simulink model "uavsimblockset_trimModel_Cularis_turbulentAtmosphere"  (Simulink 8.6)
settings: Solver=ode45  StartTime=0.0  StopTime=1  FixedStep=1/30  RelTol=1e-3
undefined symbols (not defined in the file): Earth, uavsim, WGS84
libraries: aerolibadyn x2, uavsimBlockset_DerivedAerodynamicConditions x1, uavsimBlockset_ElectricPropulsion x1, aerolibobsolete x1, aerolibtransform2 x1, uavsimblockset_vbody2vNED x1, aerolibgravity2 x1, uavsimBlockset_VectorNorm x1
settings Model: Creator=mstolle  LastModifiedBy=j.bolting
settings SolverCC: AutoInsertRateTranBlk=on
settings DataIOCC: SignalLoggingSaveFormat=Dataset
settings DebuggingCC: SolverPrmCheckMsg=none  FcnCallInpInsideContextMsg=EnableAllAsError  BusObjectLabelMismatch=error
settings ModelReferenceCC: ModelReferenceMinAlgLoopOccurrences=on
settings GRTTargetCC: CombineOutputUpdateFcns=on  GRTInterface=off
settings ConfigComp: CovSFcnEnable=off

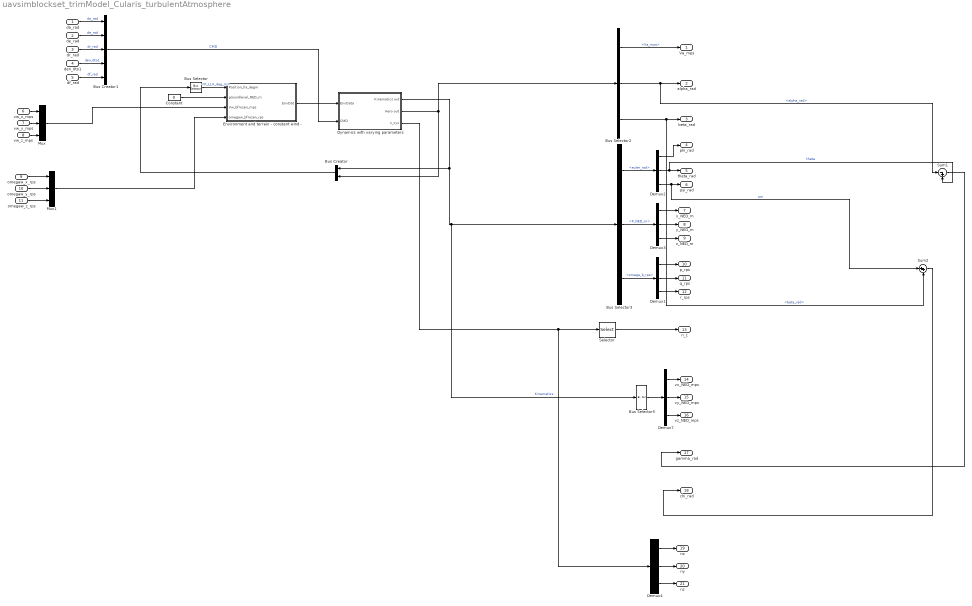
== system uavsimblockset_trimModel_Cularis_turbulentAtmosphere ==
  da_rad : Inport
  de_rad : Inport  Port=2
  dr_rad : Inport  Port=3
  den_0to1 : Inport  Port=4
  df_rad : Inport  Port=5
  vw_x_mps : Inport  Port=6  PortDimensions=1
  vw_y_mps : Inport  Port=7  PortDimensions=1
  vw_z_mps : Inport  Port=8  PortDimensions=1
  omegaw_x_rps : Inport  Port=9  PortDimensions=1
  omegaw_y_rps : Inport  Port=10  PortDimensions=1
  omegaw_z_rps : Inport  Port=11  PortDimensions=1
  Bus Creator1 : BusCreator  Inputs=5  OutDataTypeStr=Bus: CMD  NonVirtualBus=on
  Bus Creator : BusCreator  Inputs=2
  Bus Selector : BusSelector  OutputSignals=Kinematics.Position.P_LLA_deg_m
  Bus Selector2 : BusSelector  OutputSignals=Va_mps,alpha_rad,beta_rad
  Bus Selector3 : BusSelector  OutputSignals=Attitude.euler_rad,Position.P_NED_m,RotationalVelocity.omega_b_rps
  Bus Selector5 : BusSelector  OutputSignals=Velocity.Vground_NED_mps  OutputAsBus=on
  Constant : Constant  Value=0
  Demux{1..4,7} (5 alike) : Demux  Outputs=3
  Dynamics with varying parameters : Subsystem  mask{uavsim=uavsim}
      mask prompts: uavsim "Parameter structure"
  Environment and terrain - constant wind - : Subsystem  AncestorBlock=uavsimBlockset_Environment_calmAtmosphere/Environment and terrain - calm atmosphere -
  Mux : Mux  Inputs=3
  Mux1 : Mux  Inputs=3
  Selector : Selector  InputPortWidth=3  IndexOptions=Index vector (dialog)  Indices=1  OutputSizes=1
  Sum1 : Sum  Inputs=|-+
  Sum2 : Sum  Inputs=|++
  Va_mps : Outport
  alpha_rad : Outport  Port=2
  beta_rad : Outport  Port=3
  phi_rad : Outport  Port=4
  theta_rad : Outport  Port=5
  psi_rad : Outport  Port=6
  x_NED_m : Outport  Port=7
  y_NED_m : Outport  Port=8
  z_NED_m : Outport  Port=9
  p_rps : Outport  Port=10
  q_rps : Outport  Port=11
  r_rps : Outport  Port=12
  n_z : Outport  Port=13
  vx_NED_mps : Outport  Port=14
  vy_NED_mps : Outport  Port=15
  vz_NED_mps : Outport  Port=16
  gamma_rad : Outport  Port=17
  chi_rad : Outport  Port=18
  nx : Outport  Port=19
  ny : Outport  Port=20
  nz : Outport  Port=21
  wires:
  den_0to1/1 -> Bus Creator1/4  "den_0to1"
  de_rad/1 -> Bus Creator1/2  "de_rad"
  da_rad/1 -> Bus Creator1/1  "da_rad"
  dr_rad/1 -> Bus Creator1/3  "dr_rad"
  Bus Creator1/1 -> Dynamics with varying parameters/2(CMD)  "CMD"
  Environment and terrain - constant wind -/1(EnvDat) -> Dynamics with varying parameters/1(EnvData)
  df_rad/1 -> Bus Creator1/5  "df_rad"
  Bus Creator/1 -> Bus Selector/1
  Constant/1 -> Environment and terrain - constant wind -/2(groundlevel_NED_m)
  Bus Selector/1 -> Environment and terrain - constant wind -/1(Position_lla_degm)  "<P_LLA_deg_m>"
  Mux/1 -> Environment and terrain - constant wind -/3(Vw_bfrozen_mps)
  Mux1/1 -> Environment and terrain - constant wind -/4(omegaw_bfrozen_rps)
  Dynamics with varying parameters/2(Aero out) -> Bus Creator/2, Bus Selector2/1
  vw_z_mps/1 -> Mux/3
  vw_y_mps/1 -> Mux/2
  vw_x_mps/1 -> Mux/1
  omegaw_x_rps/1 -> Mux1/1
  omegaw_z_rps/1 -> Mux1/3
  omegaw_y_rps/1 -> Mux1/2
  Bus Selector3/1 -> Demux2/1  "<euler_rad>"
  Demux2/1 -> phi_rad/1
  Bus Selector3/3 -> Demux1/1  "<omega_b_rps>"
  Demux1/1 -> p_rps/1
  Demux1/2 -> q_rps/1
  Demux1/3 -> r_rps/1
  Bus Selector2/1 -> Va_mps/1  "<Va_mps>"
  Bus Selector3/2 -> Demux3/1  "<P_NED_m>"
  Demux3/1 -> x_NED_m/1
  Demux3/2 -> y_NED_m/1
  Demux3/3 -> z_NED_m/1
  Dynamics with varying parameters/3(n_xyz) -> Demux4/1, Selector/1
  Dynamics with varying parameters/1(Kinematics out) -> Bus Selector5/1, Bus Selector3/1, Bus Creator/1  "Kinematics"
  Bus Selector5/1 -> Demux7/1
  Bus Selector2/3 -> Sum2/2, beta_rad/1  "<beta_rad>"
  Bus Selector2/2 -> Sum1/1, alpha_rad/1  "<alpha_rad>"
  Demux2/2 -> theta_rad/1, Sum1/2  "theta"
  Sum1/1 -> gamma_rad/1
  Demux2/3 -> Sum2/1, psi_rad/1  "psi"
  Sum2/1 -> chi_rad/1
  Demux7/1 -> vx_NED_mps/1
  Demux7/2 -> vy_NED_mps/1
  Demux7/3 -> vz_NED_mps/1
  Selector/1 -> n_z/1
  Demux4/1 -> nx/1
  Demux4/2 -> ny/1
  Demux4/3 -> nz/1

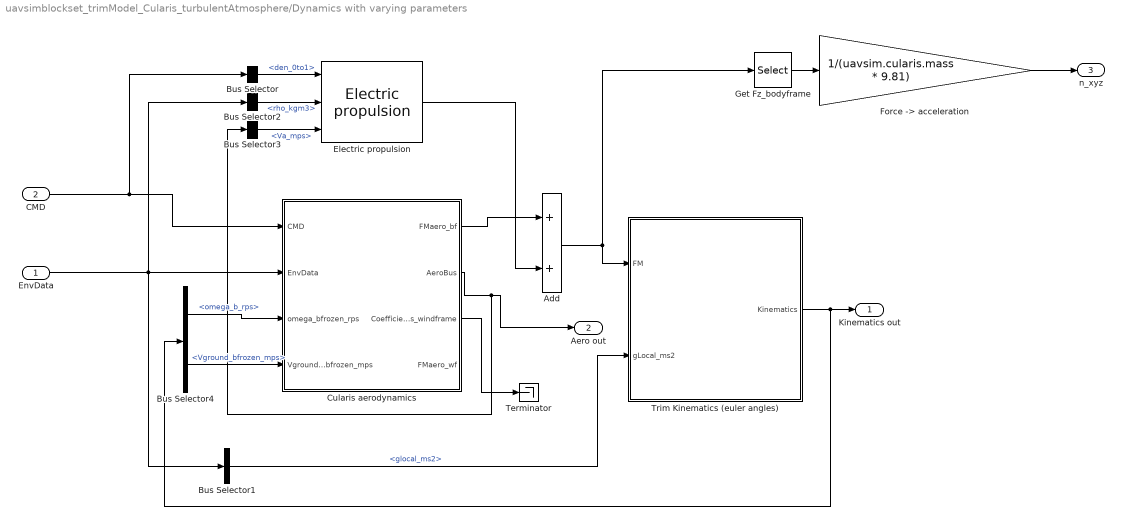
== system uavsimblockset_trimModel_Cularis_turbulentAtmosphere/Dynamics with varying parameters ==
  EnvData : Inport  OutDataTypeStr=Bus: Environment
  CMD : Inport  Port=2  OutDataTypeStr=Bus: CMD
  Add : Sum
  Bus Selector : BusSelector  OutputSignals=den_0to1
  Bus Selector1 : BusSelector  OutputSignals=glocal_ms2
  Bus Selector2 : BusSelector  OutputSignals=rho_kgm3
  Bus Selector3 : BusSelector  OutputSignals=Va_mps
  Bus Selector4 : BusSelector  OutputSignals=RotationalVelocity.omega_b_rps,Velocity.Vground_bfrozen_mps
  Cularis aerodynamics : Subsystem  AncestorBlock=uavsimBlockset_Cularis_Aerandpropulsion/Cularis aerodynamics
  Electric propulsion : uavsimBlockset_ElectricPropulsion/Electric propulsion  mask_C_prop=uavsim.cularis.C_prop  mask_S_prop=uavsim.cularis.S_prop  mask_k_motor=uavsim.cularis.k_motor
  "Force -> acceleration" : Gain  Gain=1/(uavsim.cularis.mass * 9.81)
  Get Fz_bodyframe : Selector  InputPortWidth=6  IndexOptions=Index vector (dialog)  Indices=1:3  OutputSizes=1
  Terminator : Terminator
  Trim Kinematics (euler angles) : Subsystem  AncestorBlock=uavsimblockset_TrimKinematics/Trim Kinematics (euler angles)  mask{mask_inertia=uavsim.cularis.inertiaTensor, mask_mass=uavsim.cularis.mass, mask_P0_ECEF_m=uavsim.mojaveairport_ecef_m, mask_uvw0=[15 0 0], mask_phithetapsi0=[0 0 0], mask_omega0=[0 0 0]}
      mask prompts: mask_inertia "Inertia tensor [kg * m²]"; mask_mass "Aircraft mass [kg]"; mask_P0_ECEF_m "Initial ECEF position [m]"; mask_uvw0 "Initial velocity vector, body frame [m/s]"; mask_phithetapsi0 "Initial Euler angles [rad]"; mask_omega0 "Initial body rotation rates [rad/s]"
  Kinematics out : Outport  OutDataTypeStr=Bus: Kinematics
  Aero out : Outport  Port=2  OutDataTypeStr=Bus: Aero
  n_xyz : Outport  Port=3  PortDimensions=3
  wires:
  Bus Selector4/2 -> Cularis aerodynamics/4(Vground_bfrozen_mps)  "<Vground_bfrozen_mps>"
  Bus Selector4/1 -> Cularis aerodynamics/3(omega_bfrozen_rps)  "<omega_b_rps>"
  Trim Kinematics (euler angles)/1(Kinematics) -> Kinematics out/1, Bus Selector4/1
  EnvData/1 -> Bus Selector2/1, Bus Selector1/1, Cularis aerodynamics/2(EnvData)
  Add/1 -> Get Fz_bodyframe/1, Trim Kinematics (euler angles)/1(FM)
  Cularis aerodynamics/1(FMaero_bf) -> Add/1
  Cularis aerodynamics/3(Coefficients_windframe) -> Terminator/1
  Bus Selector1/1 -> Trim Kinematics (euler angles)/2(gLocal_ms2)  "<glocal_ms2>"
  Get Fz_bodyframe/1 -> "Force -> acceleration"/1
  "Force -> acceleration"/1 -> n_xyz/1
  Bus Selector/1 -> Electric propulsion/1  "<den_0to1>"
  Bus Selector3/1 -> Electric propulsion/3  "<Va_mps>"
  Bus Selector2/1 -> Electric propulsion/2  "<rho_kgm3>"
  CMD/1 -> Bus Selector/1, Cularis aerodynamics/1(CMD)
  Cularis aerodynamics/2(AeroBus) -> Bus Selector3/1, Aero out/1
  Electric propulsion/1 -> Add/2

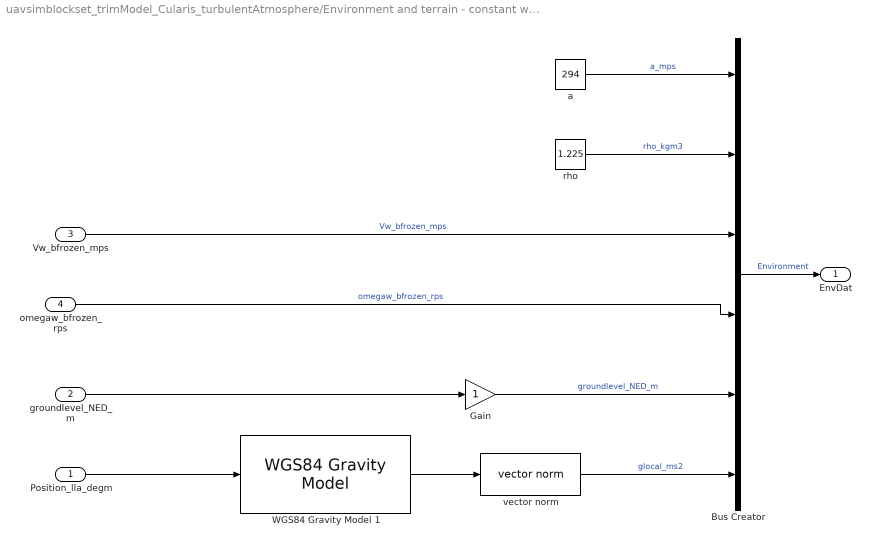
== system uavsimblockset_trimModel_Cularis_turbulentAtmosphere/Environment and terrain - constant wind - ==
  Position_lla_degm : Inport
  groundlevel_NED_m : Inport  Port=2
  Vw_bfrozen_mps : Inport  Port=3
  omegaw_bfrozen_rps : Inport  Port=4
  Bus Creator : BusCreator  Inputs=6  OutDataTypeStr=Bus: Environment  NonVirtualBus=on
  Gain : Gain
  WGS84 Gravity Model 1 : aerolibgravity2/WGS84 Gravity Model   model=WGS84 Taylor Series  units=Metric (MKS)  no_atmos=on  precessing=on  jd_loc=off  month=October  day=10  year=2004  no_centrifugal=on  action=Warning
  a : Constant  Value=294
  "rho " : Constant  Value=1.225
  vector norm : uavsimBlockset_VectorNorm/vector norm
  EnvDat : Outport  OutDataTypeStr=Bus: Environment
  wires:
  Gain/1 -> Bus Creator/5  "groundlevel_NED_m"
  omegaw_bfrozen_rps/1 -> Bus Creator/4  "omegaw_bfrozen_rps"
  vector norm/1 -> Bus Creator/6  "glocal_ms2"
  Vw_bfrozen_mps/1 -> Bus Creator/3  "Vw_bfrozen_mps"
  a/1 -> Bus Creator/1  "a_mps"
  "rho "/1 -> Bus Creator/2  "rho_kgm3"
  Bus Creator/1 -> EnvDat/1  "Environment"
  WGS84 Gravity Model 1/1 -> vector norm/1
  groundlevel_NED_m/1 -> Gain/1
  Position_lla_degm/1 -> WGS84 Gravity Model 1/1

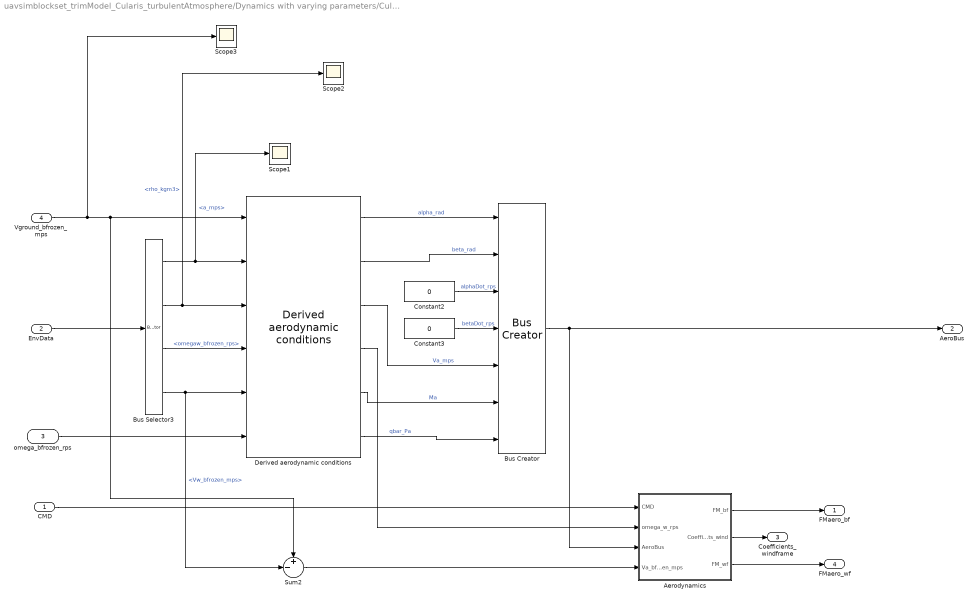
== system uavsimblockset_trimModel_Cularis_turbulentAtmosphere/Dynamics with varying parameters/Cularis aerodynamics ==
  CMD : Inport  OutDataTypeStr=Bus: CMD
  EnvData : Inport  Port=2  OutDataTypeStr=Bus: Environment
  omega_bfrozen_rps : Inport  Port=3
  Vground_bfrozen_mps : Inport  Port=4
  Aerodynamics : Subsystem
  Bus Selector3 : BusSelector  OutputSignals=a_mps,rho_kgm3,omegaw_bfrozen_rps,Vw_bfrozen_mps
  Bus Creator : BusCreator  Inputs=7
  Constant2 : Constant  Value=0
  Constant3 : Constant  Value=0
  Derived aerodynamic conditions : uavsimBlockset_DerivedAerodynamicConditions/Derived aerodynamic conditions
  Scope1 : Scope
  Scope2 : Scope
  Scope3 : Scope
  Sum2 : Sum  Inputs=+-|  SaturateOnIntegerOverflow=on  InputSameDT=on  OutDataTypeStr=Inherit: Same as first input
  FMaero_bf : Outport
  AeroBus : Outport  Port=2  OutDataTypeStr=Bus: Aero
  Coefficients_windframe : Outport  Port=3
  FMaero_wf : Outport  Port=4
  wires:
  Derived aerodynamic conditions/4 -> Aerodynamics/2(omega_w_rps)
  Sum2/1 -> Aerodynamics/4(Va_bfrozen_mps)
  Bus Creator/1 -> Aerodynamics/3(AeroBus), AeroBus/1
  Derived aerodynamic conditions/6 -> Bus Creator/7  "qbar_Pa"
  Derived aerodynamic conditions/5 -> Bus Creator/6  "Ma"
  Derived aerodynamic conditions/3 -> Bus Creator/5  "Va_mps"
  Derived aerodynamic conditions/2 -> Bus Creator/2  "beta_rad"
  Derived aerodynamic conditions/1 -> Bus Creator/1  "alpha_rad"
  Vground_bfrozen_mps/1 -> Scope3/1, Derived aerodynamic conditions/1, Sum2/1
  Constant3/1 -> Bus Creator/4  "betaDot_rps"
  Constant2/1 -> Bus Creator/3  "alphaDot_rps"
  Bus Selector3/4 -> Sum2/2, Derived aerodynamic conditions/5  "<Vw_bfrozen_mps>"
  Bus Selector3/3 -> Derived aerodynamic conditions/4  "<omegaw_bfrozen_rps>"
  Bus Selector3/2 -> Scope2/1, Derived aerodynamic conditions/3  "<rho_kgm3>"
  Bus Selector3/1 -> Scope1/1, Derived aerodynamic conditions/2  "<a_mps>"
  Aerodynamics/2(Coefficients_wind) -> Coefficients_windframe/1
  CMD/1 -> Aerodynamics/1(CMD)
  Aerodynamics/1(FM_bf) -> FMaero_bf/1
  omega_bfrozen_rps/1 -> Derived aerodynamic conditions/6
  EnvData/1 -> Bus Selector3/1
  Aerodynamics/3(FM_wf) -> FMaero_wf/1

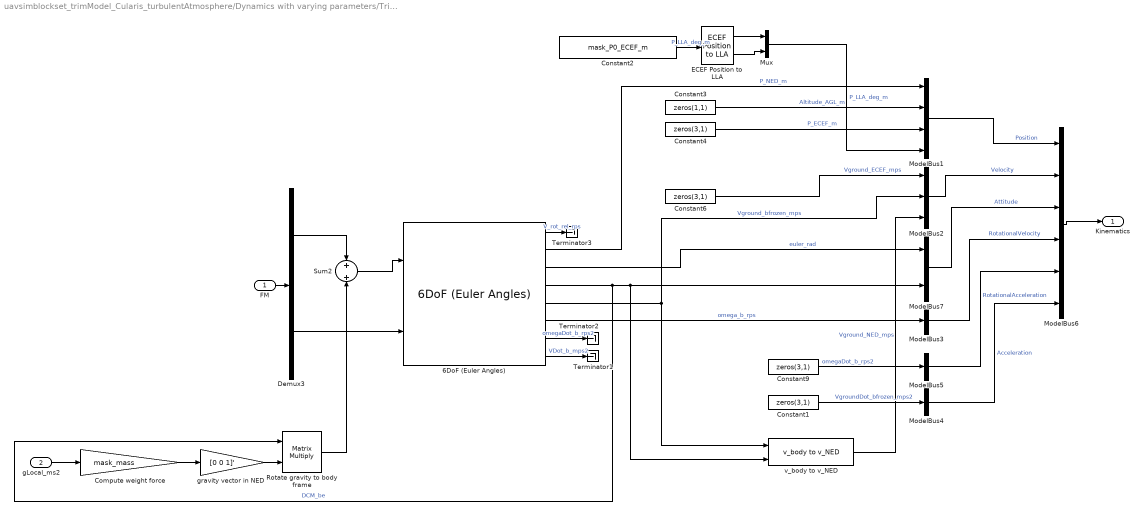
== system uavsimblockset_trimModel_Cularis_turbulentAtmosphere/Dynamics with varying parameters/Trim Kinematics (euler angles) ==
  FM : Inport
  gLocal_ms2 : Inport  Port=2
  6DoF (Euler Angles) : aerolibobsolete/6DoF (Euler Angles)  units=Metric (MKS)  mtype=Fixed  rep=Euler Angles  xme_0=mask_P0_ECEF_m  Vm_0=mask_uvw0  eul_0=mask_phithetapsi0  pm_0=mask_omega0  mass_0=mask_mass  mass_e=0.5  mass_f=2.0  inertia=mask_inertia  inertia_e=eye(3)  inertia_f=2*eye(3)  k_quat=1.0
  Compute weight force : Gain  Gain=mask_mass
  Constant{1,4,6,9} (4 alike) : Constant  Value=zeros(3,1)  SampleTime=-1
  Constant2 : Constant  Value=mask_P0_ECEF_m  SampleTime=-1
  Constant3 : Constant  Value=zeros(1,1)  SampleTime=-1
  Demux3 : Demux  Outputs=[3,3]
  ECEF Position to LLA : aerolibtransform2/ECEF Position to LLA  units=Metric (MKS)  ptype=Earth (WGS84)  F=1/298.257223563  R=6378137
  ModelBus1 : BusCreator  Inputs='P_NED_m','Altitude_AGL_m','P_ECEF_m','P_LLA_deg_m'  OutDataTypeStr=Bus: Position  NonVirtualBus=on
  ModelBus2 : BusCreator  Inputs=3  OutDataTypeStr=Bus: Velocity  NonVirtualBus=on
  ModelBus3 : BusCreator  Inputs='omega_b_rps'  OutDataTypeStr=Bus: RotationalVelocity  NonVirtualBus=on
  ModelBus4 : BusCreator  Inputs=1  OutDataTypeStr=Bus: Acceleration  NonVirtualBus=on
  ModelBus5 : BusCreator  Inputs='omegaDot_b_rps2'  OutDataTypeStr=Bus: RotationalAcceleration  NonVirtualBus=on
  ModelBus6 : BusCreator  Inputs=6  OutDataTypeStr=Bus: Kinematics
  ModelBus7 : BusCreator  Inputs='euler_rad','DCM_be'  OutDataTypeStr=Bus: Attitude  NonVirtualBus=on
  Mux : Mux  Inputs=2
  Rotate gravity to body frame : Product  Multiplication=Matrix(*)
  Sum2 : Sum  SaturateOnIntegerOverflow=on  InputSameDT=on  OutDataTypeStr=Inherit: Same as first input
  Terminator1 : Terminator
  Terminator2 : Terminator
  Terminator3 : Terminator
  gravity vector in NED : Gain  Gain=[0 0 1]'
  v_body to v_NED : uavsimblockset_vbody2vNED/v_body to v_NED
  Kinematics : Outport  OutDataTypeStr=Bus: Kinematics
  wires:
  ECEF Position to LLA/2 -> Mux/2
  ECEF Position to LLA/1 -> Mux/1
  Constant2/1 -> ECEF Position to LLA/1  "P_LLA_deg_m"
  Rotate gravity to body frame/1 -> Sum2/2
  Compute weight force/1 -> gravity vector in NED/1
  gravity vector in NED/1 -> Rotate gravity to body frame/2
  gLocal_ms2/1 -> Compute weight force/1
  v_body to v_NED/1 -> ModelBus2/3  "Vground_NED_mps"
  6DoF (Euler Angles)/1 -> Terminator3/1  "V_rot_rel_rps"
  FM/1 -> Demux3/1
  Constant9/1 -> ModelBus5/1  "omegaDot_b_rps2"
  6DoF (Euler Angles)/7 -> Terminator2/1  "omegaDot_b_rps2"
  6DoF (Euler Angles)/8 -> Terminator1/1  "VDot_b_mps2"
  Constant1/1 -> ModelBus4/1  "VgroundDot_bfrozen_mps2"
  ModelBus6/1 -> Kinematics/1
  6DoF (Euler Angles)/5 -> v_body to v_NED/1, ModelBus2/2  "Vground_bfrozen_mps"
  6DoF (Euler Angles)/2 -> ModelBus1/1  "P_NED_m"
  Mux/1 -> ModelBus1/4  "P_LLA_deg_m"
  Constant3/1 -> ModelBus1/2  "Altitude_AGL_m"
  ModelBus5/1 -> ModelBus6/5  "RotationalAcceleration"
  ModelBus2/1 -> ModelBus6/2  "Velocity"
  ModelBus3/1 -> ModelBus6/4  "RotationalVelocity"
  6DoF (Euler Angles)/3 -> ModelBus7/1  "euler_rad"
  Constant6/1 -> ModelBus2/1  "Vground_ECEF_mps"
  Demux3/2 -> 6DoF (Euler Angles)/2
  Sum2/1 -> 6DoF (Euler Angles)/1
  6DoF (Euler Angles)/6 -> ModelBus3/1  "omega_b_rps"
  6DoF (Euler Angles)/4 -> ModelBus7/2, v_body to v_NED/2, Rotate gravity to body frame/1  "DCM_be"
  Demux3/1 -> Sum2/1
  ModelBus7/1 -> ModelBus6/3  "Attitude"
  Constant4/1 -> ModelBus1/3  "P_ECEF_m"
  ModelBus1/1 -> ModelBus6/1  "Position"
  ModelBus4/1 -> ModelBus6/6  "Acceleration"

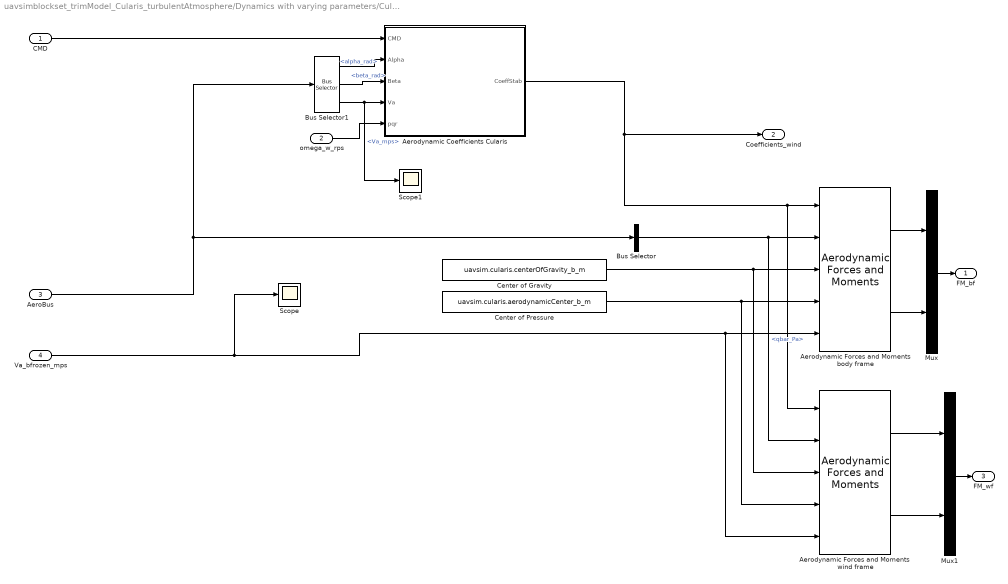
== system uavsimblockset_trimModel_Cularis_turbulentAtmosphere/Dynamics with varying parameters/Cularis aerodynamics/Aerodynamics ==
  CMD : Inport  OutDataTypeStr=Bus: CMD
  omega_w_rps : Inport  Port=2
  AeroBus : Inport  Port=3  OutDataTypeStr=Bus: Aero
  Va_bfrozen_mps : Inport  Port=4
  Aerodynamic Coefficients Cularis : Subsystem
  "Aerodynamic Forces and Moments body frame " : aerolibadyn/Aerodynamic Forces and Moments   inputAxes=Wind  outputForceAxes=Body  outputMomentAxes=Body  S=uavsim.cularis.S  b=uavsim.cularis.b  cbar=uavsim.cularis.c
  Aerodynamic Forces and Moments  wind frame : aerolibadyn/Aerodynamic Forces and Moments   inputAxes=Wind  outputForceAxes=Wind  outputMomentAxes=Wind  S=uavsim.cularis.S  b=uavsim.cularis.b  cbar=uavsim.cularis.c
  Bus Selector1 : BusSelector  OutputSignals=alpha_rad,beta_rad,Va_mps
  Bus Selector : BusSelector  OutputSignals=qbar_Pa
  Center of Gravity : Constant  Value=uavsim.cularis.centerOfGravity_b_m  SampleTime=0
  Center of Pressure : Constant  Value=uavsim.cularis.aerodynamicCenter_b_m  SampleTime=0
  Mux : Mux  Inputs=2
  Mux1 : Mux  Inputs=2
  Scope : Scope
  Scope1 : Scope
  FM_bf : Outport
  Coefficients_wind : Outport  Port=2
  FM_wf : Outport  Port=3
  wires:
  Va_bfrozen_mps/1 -> Scope/1, Aerodynamic Forces and Moments  wind frame/5, "Aerodynamic Forces and Moments body frame "/5
  omega_w_rps/1 -> Aerodynamic Coefficients Cularis/5(pqr)
  Bus Selector1/3 -> Scope1/1, Aerodynamic Coefficients Cularis/4(Va)  "<Va_mps>"
  Bus Selector1/2 -> Aerodynamic Coefficients Cularis/3(Beta)  "<beta_rad>"
  Bus Selector1/1 -> Aerodynamic Coefficients Cularis/2(Alpha)  "<alpha_rad>"
  AeroBus/1 -> Bus Selector1/1, Bus Selector/1
  Bus Selector/1 -> Aerodynamic Forces and Moments  wind frame/2, "Aerodynamic Forces and Moments body frame "/2  "<qbar_Pa>"
  Mux/1 -> FM_bf/1
  CMD/1 -> Aerodynamic Coefficients Cularis/1(CMD)
  Center of Pressure/1 -> Aerodynamic Forces and Moments  wind frame/4, "Aerodynamic Forces and Moments body frame "/4
  Center of Gravity/1 -> Aerodynamic Forces and Moments  wind frame/3, "Aerodynamic Forces and Moments body frame "/3
  "Aerodynamic Forces and Moments body frame "/1 -> Mux/1
  Aerodynamic Coefficients Cularis/1(CoeffStab) -> Coefficients_wind/1, "Aerodynamic Forces and Moments body frame "/1, Aerodynamic Forces and Moments  wind frame/1
  "Aerodynamic Forces and Moments body frame "/2 -> Mux/2
  Mux1/1 -> FM_wf/1
  Aerodynamic Forces and Moments  wind frame/1 -> Mux1/1
  Aerodynamic Forces and Moments  wind frame/2 -> Mux1/2

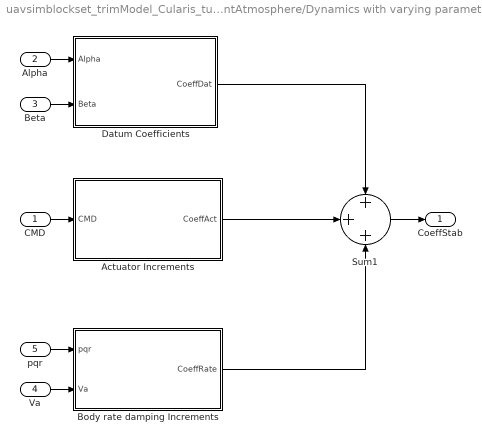
== system uavsimblockset_trimModel_Cularis_turbulentAtmosphere/Dynamics with varying parameters/Cularis aerodynamics/Aerodynamics/Aerodynamic Coefficients Cularis ==
  CMD : Inport
  Alpha : Inport  Port=2
  Beta : Inport  Port=3
  Va : Inport  Port=4
  pqr : Inport  Port=5
  Actuator Increments : Subsystem
  Body rate damping Increments : Subsystem
  Datum Coefficients : Subsystem
  Sum1 : Sum  Inputs=+++  SaturateOnIntegerOverflow=on  InputSameDT=on  OutDataTypeStr=Inherit: Same as first input
  CoeffStab : Outport
  wires:
  Datum Coefficients/1(CoeffDat) -> Sum1/1
  Sum1/1 -> CoeffStab/1
  CMD/1 -> Actuator Increments/1(CMD)
  Beta/1 -> Datum Coefficients/2(Beta)
  pqr/1 -> Body rate damping Increments/1(pqr)
  Va/1 -> Body rate damping Increments/2(Va)
  Alpha/1 -> Datum Coefficients/1(Alpha)
  Body rate damping Increments/1(CoeffRate) -> Sum1/3
  Actuator Increments/1(CoeffAct) -> Sum1/2

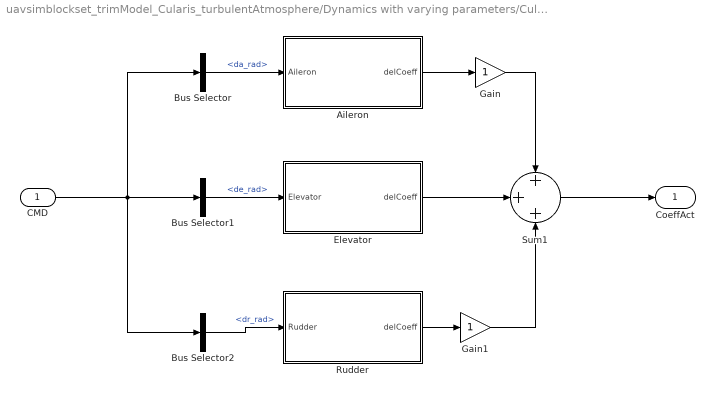
== system uavsimblockset_trimModel_Cularis_turbulentAtmosphere/Dynamics with varying parameters/Cularis aerodynamics/Aerodynamics/Aerodynamic Coefficients Cularis/Actuator Increments ==
  CMD : Inport
  Aileron : Subsystem
  Bus Selector : BusSelector  OutputSignals=da_rad
  Bus Selector1 : BusSelector  OutputSignals=de_rad
  Bus Selector2 : BusSelector  OutputSignals=dr_rad
  Elevator : Subsystem
  Gain : Gain
  Gain1 : Gain
  Rudder : Subsystem
  Sum1 : Sum  Inputs=+++  SaturateOnIntegerOverflow=on  InputSameDT=on  OutDataTypeStr=Inherit: Same as first input
  CoeffAct : Outport  InitialOutput=0
  wires:
  Elevator/1(delCoeff) -> Sum1/2
  Aileron/1(delCoeff) -> Gain/1
  Rudder/1(delCoeff) -> Gain1/1
  Sum1/1 -> CoeffAct/1
  CMD/1 -> Bus Selector/1, Bus Selector1/1, Bus Selector2/1
  Bus Selector2/1 -> Rudder/1(Rudder)  "<dr_rad>"
  Bus Selector1/1 -> Elevator/1(Elevator)  "<de_rad>"
  Bus Selector/1 -> Aileron/1(Aileron)  "<da_rad>"
  Gain/1 -> Sum1/1
  Gain1/1 -> Sum1/3

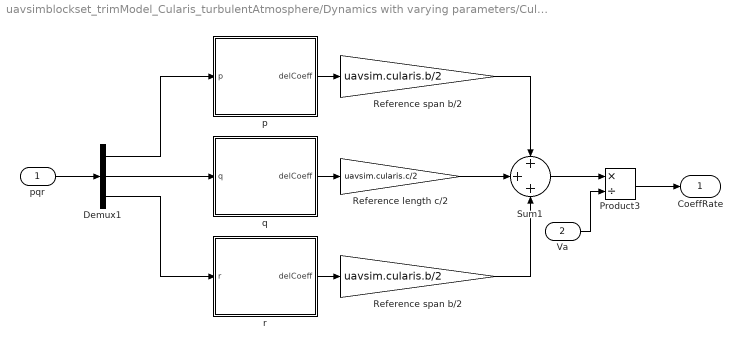
== system uavsimblockset_trimModel_Cularis_turbulentAtmosphere/Dynamics with varying parameters/Cularis aerodynamics/Aerodynamics/Aerodynamic Coefficients Cularis/Body rate damping Increments ==
  pqr : Inport
  Va : Inport  Port=2
  Demux1 : Demux  Outputs=3
  Product3 : Product  Inputs=*/  SaturateOnIntegerOverflow=on  InputSameDT=on  OutDataTypeStr=Inherit: Same as first input
  Reference length c/2 : Gain  Gain=uavsim.cularis.c/2
  Reference span b/2 : Gain  Gain=uavsim.cularis.b/2
  "Reference span b/2 " : Gain  Gain=uavsim.cularis.b/2
  Sum1 : Sum  Inputs=+++  SaturateOnIntegerOverflow=on  InputSameDT=on  OutDataTypeStr=Inherit: Same as first input
  p : Subsystem
  q : Subsystem
  r : Subsystem
  CoeffRate : Outport  InitialOutput=0
  wires:
  "Reference span b/2 "/1 -> Sum1/1
  Reference length c/2/1 -> Sum1/2
  Reference span b/2/1 -> Sum1/3
  Va/1 -> Product3/2
  Sum1/1 -> Product3/1
  Product3/1 -> CoeffRate/1
  r/1(delCoeff) -> Reference span b/2/1
  q/1(delCoeff) -> Reference length c/2/1
  p/1(delCoeff) -> "Reference span b/2 "/1
  Demux1/3 -> r/1(r)
  Demux1/2 -> q/1(q)
  Demux1/1 -> p/1(p)
  pqr/1 -> Demux1/1

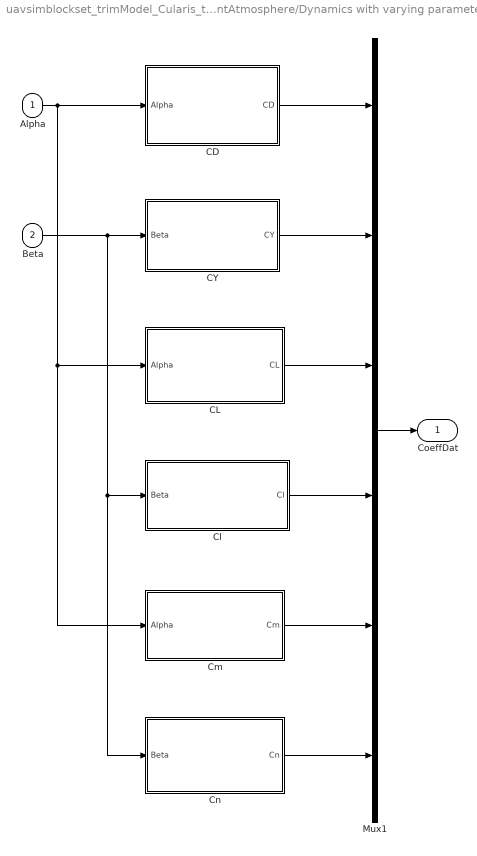
== system uavsimblockset_trimModel_Cularis_turbulentAtmosphere/Dynamics with varying parameters/Cularis aerodynamics/Aerodynamics/Aerodynamic Coefficients Cularis/Datum Coefficients ==
  Alpha : Inport
  Beta : Inport  Port=2
  CD : Subsystem
  CL : Subsystem
  CY : Subsystem
  Cl : Subsystem
  Cm : Subsystem
  Cn : Subsystem
  Mux1 : Mux  Inputs=6
  CoeffDat : Outport  InitialOutput=0
  wires:
  CL/1(CL) -> Mux1/3
  CD/1(CD) -> Mux1/1
  CY/1(CY) -> Mux1/2
  Cl/1("Cl ") -> Mux1/4
  Cm/1(Cm) -> Mux1/5
  Cn/1(Cn) -> Mux1/6
  Beta/1 -> CY/1("Beta "), Cl/1(Beta), Cn/1(Beta)
  Alpha/1 -> Cm/1(Alpha), CL/1(Alpha), CD/1(Alpha)
  Mux1/1 -> CoeffDat/1

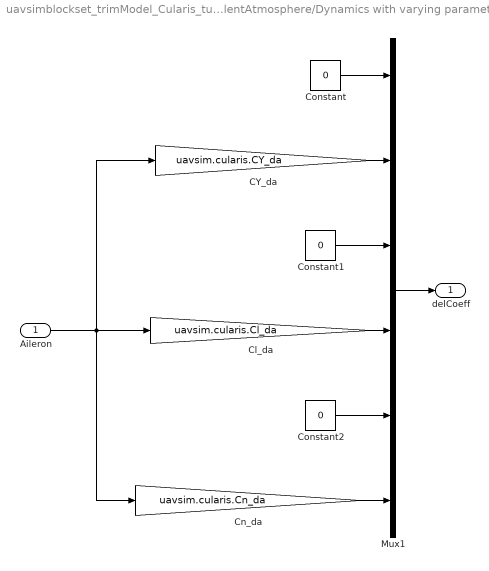
== system uavsimblockset_trimModel_Cularis_turbulentAtmosphere/Dynamics with varying parameters/Cularis aerodynamics/Aerodynamics/Aerodynamic Coefficients Cularis/Actuator Increments/Aileron ==
  Aileron : Inport
  CY_da : Gain  Gain=uavsim.cularis.CY_da
  Cl_da : Gain  Gain=uavsim.cularis.Cl_da
  Cn_da : Gain  Gain=uavsim.cularis.Cn_da
  Constant : Constant  Value=0
  Constant1 : Constant  Value=0
  Constant2 : Constant  Value=0
  Mux1 : Mux  Inputs=6
  delCoeff : Outport
  wires:
  Cn_da/1 -> Mux1/6
  Cl_da/1 -> Mux1/4
  CY_da/1 -> Mux1/2
  Mux1/1 -> delCoeff/1
  Constant/1 -> Mux1/1
  Aileron/1 -> CY_da/1, Cn_da/1, Cl_da/1
  Constant1/1 -> Mux1/3
  Constant2/1 -> Mux1/5

== system uavsimblockset_trimModel_Cularis_turbulentAtmosphere/Dynamics with varying parameters/Cularis aerodynamics/Aerodynamics/Aerodynamic Coefficients Cularis/Actuator Increments/Elevator ==
  Elevator : Inport
  CD_de : Gain  Gain=uavsim.cularis.CD_de
  CL_de : Gain  Gain=uavsim.cularis.CL_de
  Cm_de : Gain  Gain=uavsim.cularis.Cm_de
  Constant : Constant  Value=0
  Constant1 : Constant  Value=0
  Constant2 : Constant  Value=0
  Mux1 : Mux  Inputs=6
  delCoeff : Outport
  wires:
  Constant/1 -> Mux1/2
  Cm_de/1 -> Mux1/5
  CL_de/1 -> Mux1/3
  Mux1/1 -> delCoeff/1
  CD_de/1 -> Mux1/1
  Elevator/1 -> Cm_de/1, CD_de/1, CL_de/1
  Constant1/1 -> Mux1/4
  Constant2/1 -> Mux1/6

== system uavsimblockset_trimModel_Cularis_turbulentAtmosphere/Dynamics with varying parameters/Cularis aerodynamics/Aerodynamics/Aerodynamic Coefficients Cularis/Actuator Increments/Rudder ==
  Rudder : Inport
  CY_dr : Gain  Gain=uavsim.cularis.CY_dr
  Cl_dr : Gain  Gain=uavsim.cularis.Cl_dr
  Cn_dr : Gain  Gain=uavsim.cularis.Cn_dr
  Constant : Constant  Value=0
  Constant1 : Constant  Value=0
  Constant2 : Constant  Value=0
  Mux1 : Mux  Inputs=6
  delCoeff : Outport
  wires:
  Constant/1 -> Mux1/1
  Cn_dr/1 -> Mux1/6
  Cl_dr/1 -> Mux1/4
  CY_dr/1 -> Mux1/2
  Mux1/1 -> delCoeff/1
  Rudder/1 -> CY_dr/1, Cn_dr/1, Cl_dr/1
  Constant1/1 -> Mux1/3
  Constant2/1 -> Mux1/5

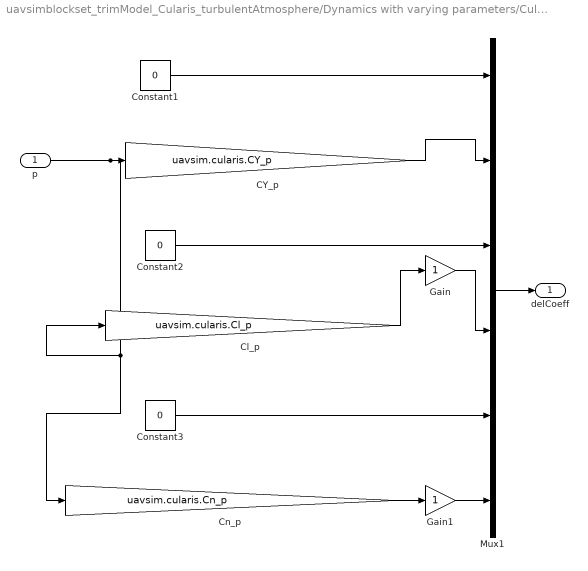
== system uavsimblockset_trimModel_Cularis_turbulentAtmosphere/Dynamics with varying parameters/Cularis aerodynamics/Aerodynamics/Aerodynamic Coefficients Cularis/Body rate damping Increments/p ==
  p : Inport
  CY_p : Gain  Gain=uavsim.cularis.CY_p
  Cl_p : Gain  Gain=uavsim.cularis.Cl_p
  Cn_p : Gain  Gain=uavsim.cularis.Cn_p
  Constant1 : Constant  Value=0
  Constant2 : Constant  Value=0
  Constant3 : Constant  Value=0
  Gain : Gain
  Gain1 : Gain
  Mux1 : Mux  Inputs=6
  delCoeff : Outport
  wires:
  p/1 -> Cn_p/1, Cl_p/1, CY_p/1
  CY_p/1 -> Mux1/2
  Constant1/1 -> Mux1/1
  Cn_p/1 -> Gain1/1
  Cl_p/1 -> Gain/1
  Mux1/1 -> delCoeff/1
  Constant2/1 -> Mux1/3
  Constant3/1 -> Mux1/5
  Gain/1 -> Mux1/4
  Gain1/1 -> Mux1/6

== system uavsimblockset_trimModel_Cularis_turbulentAtmosphere/Dynamics with varying parameters/Cularis aerodynamics/Aerodynamics/Aerodynamic Coefficients Cularis/Body rate damping Increments/q ==
  q : Inport
  CD_q : Gain  Gain=uavsim.cularis.CD_q
  CL_q : Gain  Gain=uavsim.cularis.CL_q
  Cm_q : Gain  Gain=uavsim.cularis.Cm_q
  Constant1 : Constant  Value=0
  Constant2 : Constant  Value=0
  Constant3 : Constant  Value=0
  Mux1 : Mux  Inputs=6
  delCoeff : Outport
  wires:
  Cm_q/1 -> Mux1/5
  CL_q/1 -> Mux1/3
  CD_q/1 -> Mux1/1
  Constant1/1 -> Mux1/2
  q/1 -> Cm_q/1, CL_q/1, CD_q/1
  Mux1/1 -> delCoeff/1
  Constant2/1 -> Mux1/4
  Constant3/1 -> Mux1/6

== system uavsimblockset_trimModel_Cularis_turbulentAtmosphere/Dynamics with varying parameters/Cularis aerodynamics/Aerodynamics/Aerodynamic Coefficients Cularis/Body rate damping Increments/r ==
  r : Inport
  CY_r : Gain  Gain=uavsim.cularis.CY_r
  Cl_r : Gain  Gain=uavsim.cularis.Cl_r
  Cn_r : Gain  Gain=uavsim.cularis.Cn_r
  Constant1 : Constant  Value=0
  Constant2 : Constant  Value=0
  Constant3 : Constant  Value=0
  Mux1 : Mux  Inputs=6
  delCoeff : Outport
  wires:
  Cn_r/1 -> Mux1/6
  Cl_r/1 -> Mux1/4
  CY_r/1 -> Mux1/2
  Constant1/1 -> Mux1/1
  r/1 -> Cn_r/1, Cl_r/1, CY_r/1
  Mux1/1 -> delCoeff/1
  Constant2/1 -> Mux1/3
  Constant3/1 -> Mux1/5

== system uavsimblockset_trimModel_Cularis_turbulentAtmosphere/Dynamics with varying parameters/Cularis aerodynamics/Aerodynamics/Aerodynamic Coefficients Cularis/Datum Coefficients/CD ==
  Alpha : Inport
  CD_0 : Constant  Value=uavsim.cularis.CD_0
  CL_0 : Constant  Value=uavsim.cularis.CL_0
  CL_alpha : Gain  Gain=uavsim.cularis.CL_alpha
  Product : Product  RndMeth=Zero
  Sum1 : Sum  Inputs=|++
  Sum2 : Sum  Inputs=|++
  sec. order lift contribution : Gain  Gain=1/(pi*uavsim.cularis.oswald*uavsim.cularis.AR )
  CD : Outport
  wires:
  CL_alpha/1 -> Sum2/2
  Alpha/1 -> CL_alpha/1
  Sum1/1 -> CD/1
  CD_0/1 -> Sum1/2
  sec. order lift contribution/1 -> Sum1/1
  Product/1 -> sec. order lift contribution/1
  Sum2/1 -> Product/1, Product/2
  CL_0/1 -> Sum2/1

== system uavsimblockset_trimModel_Cularis_turbulentAtmosphere/Dynamics with varying parameters/Cularis aerodynamics/Aerodynamics/Aerodynamic Coefficients Cularis/Datum Coefficients/CL ==
  note: CL_0
  Alpha : Inport
  1 : Constant  Value=uavsim.cularis.CL_0
  CL_alpha : Gain  Gain=uavsim.cularis.CL_alpha
  Sum2 : Sum  Inputs=|++
  CL : Outport
  wires:
  Sum2/1 -> CL/1
  CL_alpha/1 -> Sum2/1
  Alpha/1 -> CL_alpha/1
  1/1 -> Sum2/2

== system uavsimblockset_trimModel_Cularis_turbulentAtmosphere/Dynamics with varying parameters/Cularis aerodynamics/Aerodynamics/Aerodynamic Coefficients Cularis/Datum Coefficients/CY ==
  "Beta " : Inport
  "CY_0 " : Constant  Value=uavsim.cularis.CY_0
  CY_beta : Gain  Gain=uavsim.cularis.CY_beta  SaturateOnIntegerOverflow=on  OutDataTypeStr=Inherit: Same as input  ParamDataTypeStr=Inherit: Same as input
  Sum : Sum  Inputs=|++
  CY : Outport
  wires:
  "CY_0 "/1 -> Sum/1
  CY_beta/1 -> Sum/2
  Sum/1 -> CY/1
  "Beta "/1 -> CY_beta/1

== system uavsimblockset_trimModel_Cularis_turbulentAtmosphere/Dynamics with varying parameters/Cularis aerodynamics/Aerodynamics/Aerodynamic Coefficients Cularis/Datum Coefficients/Cl ==
  Beta : Inport
  "Cl_0 " : Constant  Value=uavsim.cularis.Cl_0
  Cl_beta : Gain  Gain=uavsim.cularis.Cl_beta  SaturateOnIntegerOverflow=on  OutDataTypeStr=Inherit: Same as input  ParamDataTypeStr=Inherit: Same as input
  Sum1 : Sum  Inputs=|++
  "Cl " : Outport
  wires:
  Beta/1 -> Cl_beta/1
  Sum1/1 -> "Cl "/1
  "Cl_0 "/1 -> Sum1/2
  Cl_beta/1 -> Sum1/1

== system uavsimblockset_trimModel_Cularis_turbulentAtmosphere/Dynamics with varying parameters/Cularis aerodynamics/Aerodynamics/Aerodynamic Coefficients Cularis/Datum Coefficients/Cm ==
  Alpha : Inport
  Cm_0 : Constant  Value=uavsim.cularis.Cm_0
  Cm_alpha : Gain  Gain=uavsim.cularis.Cm_alpha  SaturateOnIntegerOverflow=on  OutDataTypeStr=Inherit: Same as input  ParamDataTypeStr=Inherit: Same as input
  Sum2 : Sum  Inputs=|++
  Cm : Outport
  wires:
  Alpha/1 -> Cm_alpha/1
  Cm_alpha/1 -> Sum2/1
  Sum2/1 -> Cm/1
  Cm_0/1 -> Sum2/2

== system uavsimblockset_trimModel_Cularis_turbulentAtmosphere/Dynamics with varying parameters/Cularis aerodynamics/Aerodynamics/Aerodynamic Coefficients Cularis/Datum Coefficients/Cn ==
  Beta : Inport
  Cn_0 : Constant  Value=uavsim.cularis.Cn_0
  Cn_beta : Gain  Gain=uavsim.cularis.Cn_beta  SaturateOnIntegerOverflow=on  OutDataTypeStr=Inherit: Same as input  ParamDataTypeStr=Inherit: Same as input
  Sum3 : Sum  Inputs=|++
  Cn : Outport
  wires:
  Beta/1 -> Cn_beta/1
  Cn_beta/1 -> Sum3/1
  Sum3/1 -> Cn/1
  Cn_0/1 -> Sum3/2
